simulink model "sampleModel237"  (R2021b)
settings: Solver=VariableStepAuto  StartTime=0.0  StopTime=10.0  RelTol=1e-3
undefined symbols (not defined in the file or in its folder): Newton, Raphson
libraries: simulink x2
settings Model: Creator=user  LastModifiedBy=user

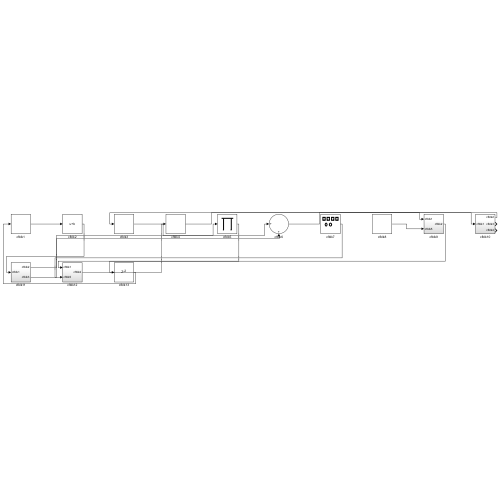
[thumbnail: Simulink's stored preview of the top-level diagram]
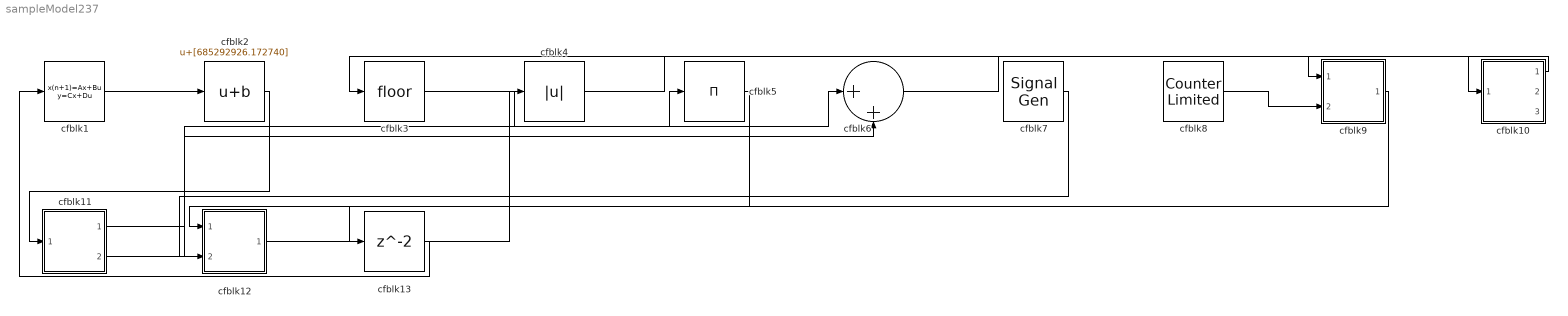
== system sampleModel237 ==
  cfblk1 : DiscreteStateSpace
  cfblk10 : Subsystem
  cfblk11 : Subsystem
  cfblk12 : Subsystem
  cfblk13 : Delay  SampleTime=1
  cfblk2 : Bias  Bias=[685292926.172740]
  cfblk3 : Rounding
  cfblk4 : Abs
  cfblk5 : Product  Inputs=*
  cfblk6 : Sum  Inputs=|++
  cfblk7 : SignalGenerator  Amplitude=[-287684201.029007]
  cfblk8 : simulink/Sources/Counter Limited  uplimit=[291.000000]  tsamp=-1
  cfblk9 : Subsystem
  wires:
  cfblk3/1 -> cfblk5/1
  cfblk1/1 -> cfblk2/1
  cfblk9/1(cfblk2) -> cfblk12/1(cfblk1)
  cfblk6/1 -> cfblk9/1(cfblk1)
  cfblk4/1 -> cfblk10/1(cfblk1)
  cfblk10/1(cfblk2) -> cfblk3/1
  cfblk7/1 -> cfblk12/2(cfblk5)
  cfblk12/1(cfblk2) -> cfblk4/1
  cfblk8/1 -> cfblk9/2(cfblk5)
  cfblk2/1 -> cfblk11/1(cfblk1)
  cfblk11/1(cfblk2) -> cfblk6/1
  cfblk11/2(cfblk3) -> cfblk6/2
  cfblk5/1 -> cfblk13/1
  cfblk13/1 -> cfblk1/1

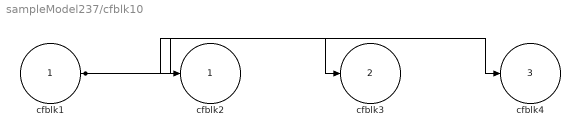
== system sampleModel237/cfblk10 ==
  cfblk1 : Inport
  cfblk2 : Outport
  cfblk3 : Outport  Port=2
  cfblk4 : Outport  Port=3
  wires:
  cfblk1/1 -> cfblk4/1, cfblk2/1, cfblk3/1

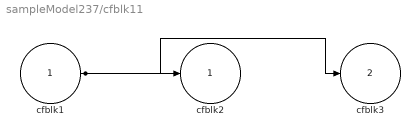
== system sampleModel237/cfblk11 ==
  cfblk1 : Inport
  cfblk2 : Outport
  cfblk3 : Outport  Port=2
  wires:
  cfblk1/1 -> cfblk2/1, cfblk3/1

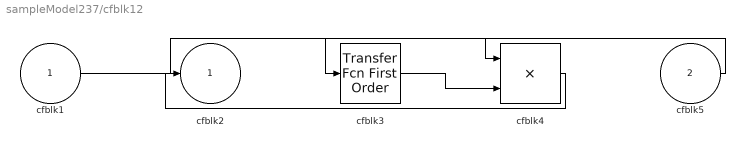
== system sampleModel237/cfblk12 ==
  cfblk1 : Inport
  cfblk5 : Inport  Port=2
  cfblk3 : simulink/Discrete/Transfer Fcn First Order  PoleZ=0.95  ICPrevOutput=0.0  DoSatur=off
  cfblk4 : Product  Inputs=**
  cfblk2 : Outport
  wires:
  cfblk1/1 -> cfblk4/1
  cfblk4/1 -> cfblk2/1
  cfblk5/1 -> cfblk3/1
  cfblk3/1 -> cfblk4/2

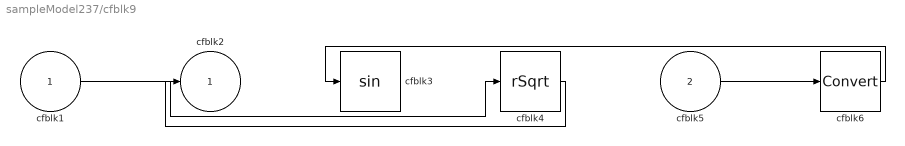
== system sampleModel237/cfblk9 ==
  cfblk1 : Inport
  cfblk5 : Inport  Port=2
  cfblk3 : Trigonometry
  cfblk4 : Sqrt  Operator=rSqrt  AlgorithmType=Newton-Raphson  SaturateOnIntegerOverflow=on
  cfblk6 : DataTypeConversion
  cfblk2 : Outport
  wires:
  cfblk1/1 -> cfblk4/1
  cfblk4/1 -> cfblk2/1
  cfblk5/1 -> cfblk6/1
  cfblk6/1 -> cfblk3/1
